simulink model "jc_3"  (R2020a)
settings: Solver=ode4  StartTime=0.0  StopTime=inf  FixedStep=0.001  RelTol=1e-3
undefined symbols (not defined in the file or in its folder): National_Instruments, PCIe
libraries: sldrtlib x3
settings Model: SimulationMode=external  ExtModeTrigDuration=60000  ExtModeArchiveMode=auto  ExtModeArchiveFileName=data  ExtModeArchiveDirName=E:\work\me-clab2\Lab02  ExtModeAddSuffixToVar=on  Creator=me-clab2  LastModifiedBy=me-clab2
settings RTWCC: Description=Simulink Desktop Real-Time  SystemTargetFile=sldrt.tlc  TemplateMakefile=sldrt.tmf  RTWCompilerOptimization=on
settings CodeAppCC: MaxIdLength=95
settings SimulinkDesktopRealTimeCC: TargetPreCompLibLocation=C:\Program Files\MATLAB\R2020a\toolbox\sldrt\lib\win64

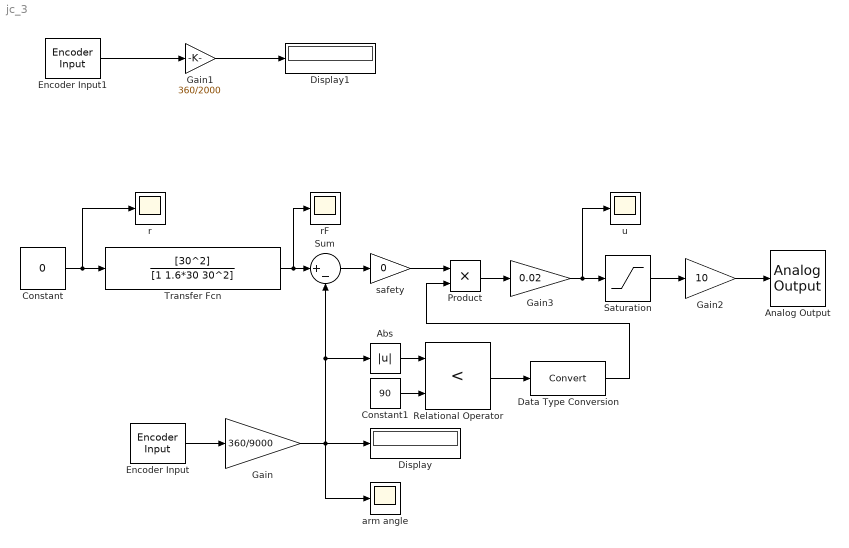
== system jc_3 ==
  Abs : Abs
  Analog Output : sldrtlib/Analog Output  SampleTime=0.001  MaxMissedTicks=10  ShowMissedTicks=off  YieldWhenWaiting=off  DrvName=National_Instruments/PCIe-6321  DrvAddress=4294967295  DrvOptions=[0 0 0 2 2 2 2]  Channels=[2]  RangeMode=1  VoltRange=1  InitialValue=0  FinalValue=0
      settings: AttributesFormatString=National Instruments\nPCIe-6321 [auto]
  Constant : Constant  Value=0
  Constant1 : Constant  Value=90
  Data Type Conversion : DataTypeConversion
  Display : Display
  Display1 : Display
  Encoder Input : sldrtlib/Encoder Input  SampleTime=0.001  MaxMissedTicks=10  ShowMissedTicks=off  YieldWhenWaiting=off  DrvName=National_Instruments/PCIe-6321  DrvAddress=4294967295  DrvOptions=[0 0 0 2 2 2 2]  Channels=[1]  QuadMode=3  IndexPulse=1  InputFilter=Inf  DataType=1
      settings: AttributesFormatString=National Instruments\nPCIe-6321 [auto]
  Encoder Input1 : sldrtlib/Encoder Input  SampleTime=0.001  MaxMissedTicks=10  ShowMissedTicks=off  YieldWhenWaiting=off  DrvName=National_Instruments/PCIe-6321  DrvAddress=4294967295  DrvOptions=[0 0 0 2 2 2 2]  Channels=[2]  QuadMode=3  IndexPulse=1  InputFilter=Inf  DataType=1
      settings: AttributesFormatString=National Instruments\nPCIe-6321 [auto]
  Gain : Gain  Gain=360/9000
  Gain1 : Gain  Gain=360/2000
  Gain2 : Gain  Gain=10
  Gain3 : Gain  Gain=0.02
  Product : Product
  Relational Operator : RelationalOperator  Operator=<  OutDataTypeStr=boolean  RndMeth=Simplest
  Saturation : Saturate  UpperLimit=1  LowerLimit=-1
  Sum : Sum  Inputs=|+-
  Transfer Fcn : TransferFcn  Numerator=[30^2]  Denominator=[1 1.6*30 30^2]
  arm angle : Scope
  r : Scope
  rF : Scope
  safety : Gain  Gain=0
  u : Scope
  wires:
  Encoder Input1/1 -> Gain1/1
  Encoder Input/1 -> Gain/1
  Gain1/1 -> Display1/1
  Gain/1 -> Display/1, arm angle/1, Abs/1, Sum/2
  Gain2/1 -> Analog Output/1
  Saturation/1 -> Gain2/1
  Transfer Fcn/1 -> rF/1, Sum/1
  Constant/1 -> Transfer Fcn/1, r/1
  Sum/1 -> safety/1
  Gain3/1 -> u/1, Saturation/1
  safety/1 -> Product/1
  Product/1 -> Gain3/1
  Abs/1 -> Relational Operator/1
  Constant1/1 -> Relational Operator/2
  Relational Operator/1 -> Data Type Conversion/1
  Data Type Conversion/1 -> Product/2
